simulink model "EX62a"  (R2014b)
settings: Solver=FixedStepDiscrete  StartTime=0.0  StopTime=.02  RelTol=1e-3
libraries: commrandsrc2 x1
settings Model: Creator=Silage  LastModifiedBy=Silage
settings DataIOCC: SignalLoggingSaveFormat=ModelDataLogs
settings OptimizationCC: ExpressionDepthLimit=2147483647
settings DebuggingCC: UnderspecifiedInitializationDetection=Classic  MergeDetectMultiDrivingBlocksExec=none  FcnCallInpInsideContextMsg=EnableAllAsWarning  StateNameClashWarn=warning
settings GRTTargetCC: CombineOutputUpdateFcns=off  GRTInterface=on

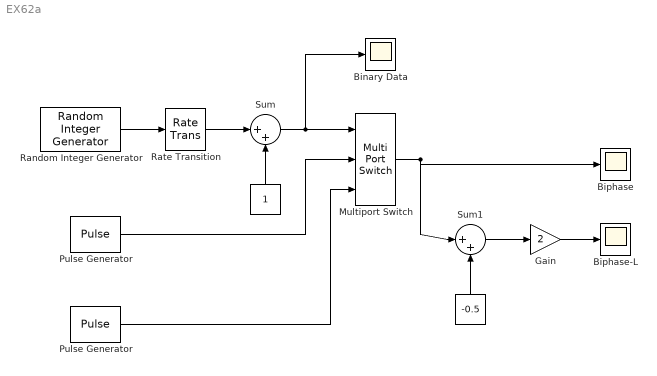
== system EX62a ==
  " " : Constant
  "   " : Constant  Value=-0.5
  Binary Data : Scope
      settings: SaveName=ScopeData2
  Biphase : Scope
      settings: YMin=-1.5  YMax=1.5
  Biphase-L : Scope
      settings: YMin=-1.5  YMax=1.5
  Gain : Gain  Gain=2
  Multiport Switch : MultiPortSwitch  Inputs=2
  Pulse Generator : DiscretePulseGenerator  Period=50  PulseWidth=25  PhaseDelay=25  SampleTime=2e-5
  "Pulse Generator " : DiscretePulseGenerator  Period=50  PulseWidth=25  SampleTime=2e-5
  Random Integer Generator : commrandsrc2/Random Integer Generator  mul=2  seed=randseed  Ts=1e-3  frameBased=off  sampPerFrame=1  orient=on  outDataType=double
  Rate Transition : RateTransition  OutPortSampleTime=2e-5
  Sum : Sum  Inputs=|++
  Sum1 : Sum  Inputs=|++
  wires:
  Random Integer Generator/1 -> Rate Transition/1
  Rate Transition/1 -> Sum/1
  " "/1 -> Sum/2
  Sum/1 -> Multiport Switch/1, Binary Data/1
  Pulse Generator/1 -> Multiport Switch/2
  "Pulse Generator "/1 -> Multiport Switch/3
  Multiport Switch/1 -> Biphase/1, Sum1/1
  "   "/1 -> Sum1/2
  Sum1/1 -> Gain/1
  Gain/1 -> Biphase-L/1
